simulink model "Traffic_Moore"  (R2020a)
settings: Solver=FixedStepDiscrete  StartTime=0.0  StopTime=150  FixedStep=0.1  RelTol=1e-3  EnableMultiTasking=on
undefined symbols (not defined in the file): DiscIntNeverNeededParam
libraries: simulink x1
settings Model: Creator=kiran  LastModifiedBy=kiran

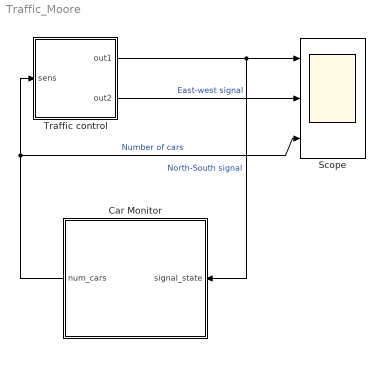
== system Traffic_Moore ==
  Car Monitor : Subsystem
  Scope : Scope  NumInputPorts=3
  Traffic control : Stateflow chart  TreatAsAtomicUnit=on
  wires:
  Traffic control/1(out1) -> Scope/1, Car Monitor/1(signal_state)  "North-South signal"
  Car Monitor/1(num_cars) -> Traffic control/1(sens), Scope/3  "Number of cars"
  Traffic control/2(out2) -> Scope/2  "East-west signal"

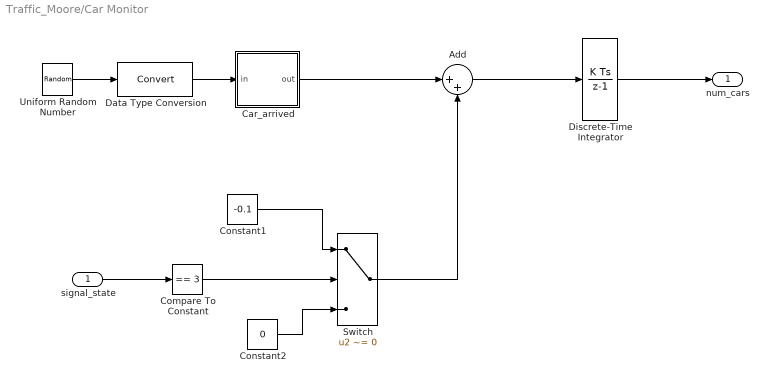
== system Traffic_Moore/Car Monitor ==
  signal_state : Inport
  Add : Sum  Inputs=|++
  Car_arrived : Stateflow chart  TreatAsAtomicUnit=on
  Compare To Constant : simulink/Logic and Bit Operations/Compare To Constant  relop===  const=3  OutDataTypeStr=boolean  ZeroCross=off
  Constant1 : Constant  Value=-0.1
  Constant2 : Constant  Value=0
  Data Type Conversion : DataTypeConversion
  Discrete-Time Integrator : DiscreteIntegrator  SampleTime=-1  LimitOutput=on  LowerSaturationLimit=0  ICPrevOutput=DiscIntNeverNeededParam  ICPrevScaledInput=DiscIntNeverNeededParam
  Switch : Switch  Criteria=u2 ~= 0
  Uniform Random Number : UniformRandomNumber  Minimum=0  Maximum=100  Seed=177836  SampleTime=0
  num_cars : Outport  VectorParamsAs1DForOutWhenUnconnected=off
  wires:
  Data Type Conversion/1 -> Car_arrived/1(in)
  signal_state/1 -> Compare To Constant/1
  Add/1 -> Discrete-Time Integrator/1
  Constant1/1 -> Switch/1
  Discrete-Time Integrator/1 -> num_cars/1
  Uniform Random Number/1 -> Data Type Conversion/1
  Switch/1 -> Add/2
  Constant2/1 -> Switch/3
  Compare To Constant/1 -> Switch/2
  Car_arrived/1(out) -> Add/1

== stateflow chart Traffic_Moore/Car Monitor/Car_arrived ==
  (default) -> (junction 2) : {out = in > 98;}
  data: in input int8; out output double

== stateflow chart Traffic_Moore/Traffic control ==
  state StopForTraffic
    out1 = RED;
    out2 = GREEN;
  state Stop
    out1 = RED;
    out2 = GREEN;
  state StopToGo
    out1 = RED;
    out2 = YELLOW;
  state GoToStop
    out1 = YELLOW;
    out2 = RED;
  state Go
    out1 = GREEN;
    out2 = RED;
  Stop -> StopForTraffic : after(20,tick)
  StopForTraffic -> StopToGo : [sens]
  (default) -> Stop
  GoToStop -> Stop : after (3,tick)
  StopToGo -> Go : after(3,tick)
  Go -> GoToStop : after(10,tick)
  data: GREEN constant double =3; YELLOW constant double =2; RED constant double =1; sens input; out1 output; out2 output
